simulink model "Prova_es2_sim_MIK"  (R2022b)
settings: Solver=VariableStepAuto  StartTime=0.0  StopTime=10.0  RelTol=1e-3
values from neighbouring files (symbols this model uses):
  A0 = sysC_d.A(2,2)-(L*sysC_d.A(1,2))    [Prova_es2.m]    (also in Prova_es2_MIK.m = sysC_d.A-(L*sysC_d.C))
  B0 = [sysC_d.B(2)-(L*sysC_d.B(1)) (A0*L)-sysC_d.A(2,1)-(L*sysC_d.A(1,1))]    [Prova_es2.m]    (also in Prova_es2_MIK.m = [sysC_d.B L])
  C0 = [0;1]    [Prova_es2.m]    (also in Prova_es2_MIK.m = eye(2))
  D0 = [0 1; 0 L]    [Prova_es2.m]    (also in Prova_es2_MIK.m = zeros(2))
  Nu = X(3)    [Prova_es2.m]    (also in Prova_es2_MIK.m)
  Nx = X(1:2)    [Prova_es2.m]    (also in Prova_es2_MIK.m)
  T = 0.01    [Prova_es2.m]    (also in Prova_es2_MIK.m)
undefined symbols (not defined in the file or in its folder): den, DiscIntNeverNeededParam, intg, num
settings Model: Creator=marcoverri  LastModifiedBy=marcoverri

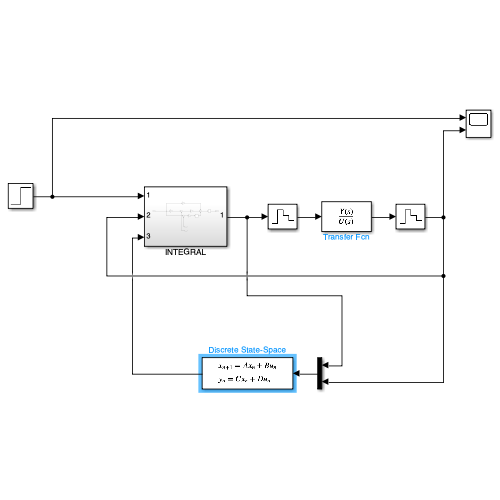
[thumbnail: Simulink's stored preview of the top-level diagram]
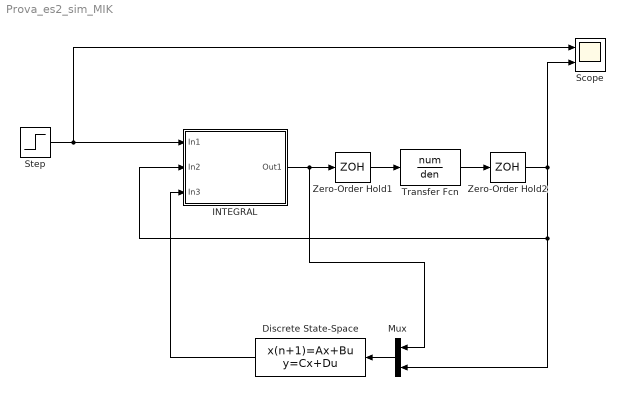
== system Prova_es2_sim_MIK ==
  Discrete State-Space : DiscreteStateSpace  A=A0  B=B0  C=C0  D=D0  SampleTime=T
  INTEGRAL : Subsystem
  Mux : Mux  Inputs=2
  Scope : Scope  NumInputPorts=2
  Step : Step  SampleTime=T
  Transfer Fcn : TransferFcn  Numerator=num  Denominator=den
  Zero-Order Hold1 : ZeroOrderHold  SampleTime=T
  Zero-Order Hold2 : ZeroOrderHold  SampleTime=T
  wires:
  Step/1 -> INTEGRAL/1(In1), Scope/1
  Mux/1 -> Discrete State-Space/1
  INTEGRAL/1(Out1) -> Mux/1, Zero-Order Hold1/1
  Zero-Order Hold2/1 -> Mux/2, INTEGRAL/2(In2), Scope/2
  Transfer Fcn/1 -> Zero-Order Hold2/1
  Zero-Order Hold1/1 -> Transfer Fcn/1
  Discrete State-Space/1 -> INTEGRAL/3(In3)

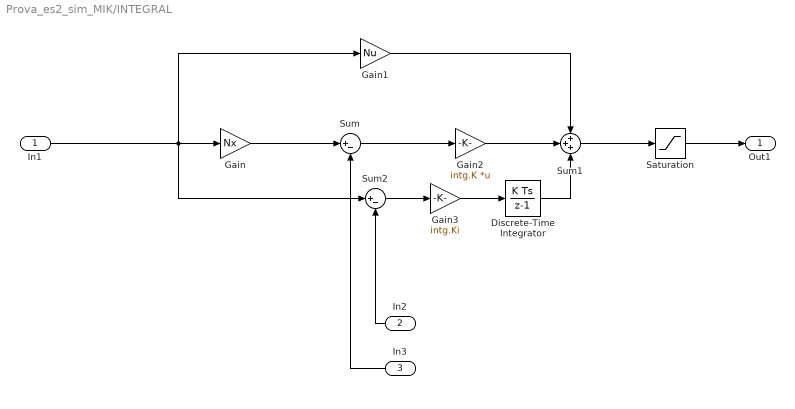
== system Prova_es2_sim_MIK/INTEGRAL ==
  In1 : Inport
  In2 : Inport  Port=2
  In3 : Inport  Port=3
  Discrete-Time Integrator : DiscreteIntegrator  SampleTime=T  ICPrevOutput=DiscIntNeverNeededParam  ICPrevScaledInput=DiscIntNeverNeededParam
  Gain : Gain  Gain=Nx
  Gain1 : Gain  Gain=Nu
  Gain2 : Gain  Gain=intg.K  Multiplication=Matrix(K*u)
  Gain3 : Gain  Gain=intg.Ki
  Saturation : Saturate  UpperLimit=10  LowerLimit=-10
  Sum : Sum  Inputs=|+-
  Sum1 : Sum  Inputs=+++
  Sum2 : Sum  Inputs=|+-
  Out1 : Outport
  wires:
  Gain/1 -> Sum/1
  Sum/1 -> Gain2/1
  Gain2/1 -> Sum1/2
  Gain1/1 -> Sum1/1
  In1/1 -> Sum2/1, Gain1/1, Gain/1
  Sum1/1 -> Saturation/1
  Saturation/1 -> Out1/1
  Discrete-Time Integrator/1 -> Sum1/3
  Gain3/1 -> Discrete-Time Integrator/1
  Sum2/1 -> Gain3/1
  In2/1 -> Sum2/2
  In3/1 -> Sum/2
